simulink model "computedTorquePD"  (R2016a)
settings: Solver=ode45  StartTime=0.0  StopTime=5  RelTol=1e-3
undefined symbols (not defined in the file): ADAMS_cwd, ADAMS_exec, ADAMS_host, ADAMS_init, ADAMS_inputs, ADAMS_outputs, ADAMS_prefix, ADAMS_static, ADAMS_sysdir
settings Model: Creator=admin  LastModifiedBy=Aniket
settings SolverCC: ZeroCrossControl=DisableAll  AlgebraicLoopSolver=LineSearch
settings DataIOCC: LimitDataPoints=on  SaveFormat=Array
settings DebuggingCC: AlgebraicLoopMsg=none
settings HardwareCC: ProdBitPerPointer=32  ProdLargestAtomicFloat=None  ProdIntDivRoundTo=Undefined  ProdEndianess=Unspecified  ProdWordSize=32  ProdHWDeviceType=32-bit Generic
settings ModelReferenceCC: PropagateSignalLabelsOutOfModel=off
settings ConfigComp: CovModelRefEnable=Off

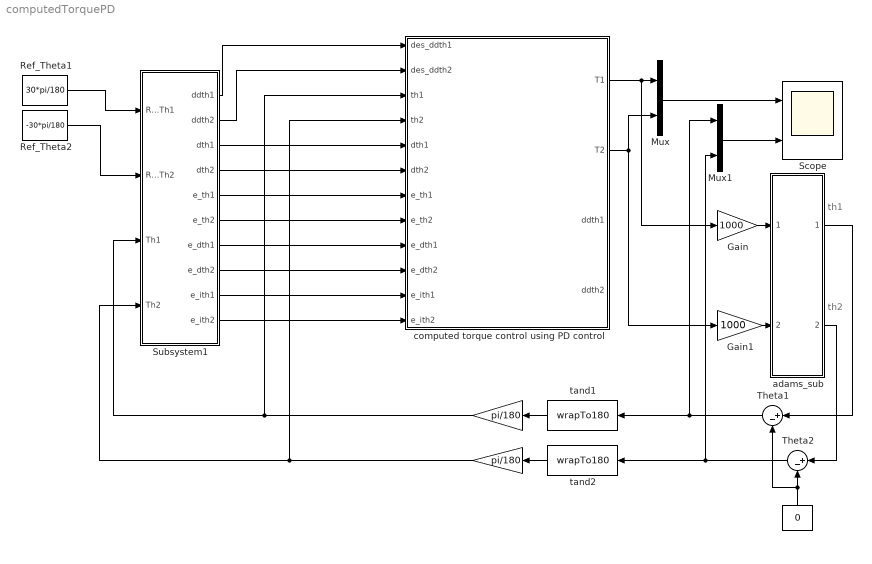
== system computedTorquePD ==
  note: th1
  note: th2
  " " : Constant  Value=0  SampleTime=-1
  "  " : Gain  Gain=pi/180
  "   " : Gain  Gain=pi/180
  Gain : Gain  Gain=1000
  Gain1 : Gain  Gain=1000
  Mux : Mux  Inputs=2
  Mux1 : Mux  Inputs=2
  Ref_Theta1 : Constant  Value=30*pi/180  SampleTime=-1
  Ref_Theta2 : Constant  Value=-30*pi/180  SampleTime=-1
  Scope : Scope  NumInputPorts=2
  Subsystem1 : Subsystem
  Theta1 : Sum  Inputs=|+-
  Theta2 : Sum  Inputs=|+-
  adams_sub : Subsystem
  computed torque control using PD control : MATLAB Function  TreatAsAtomicUnit=on
  tand1 : MATLABFcn  MATLABFcn=wrapTo180
  tand2 : MATLABFcn  MATLABFcn=wrapTo180
  wires:
  Gain/1 -> adams_sub/1("Torque_rear ")
  computed torque control using PD control/1(T1) -> Mux/1, Gain/1
  Ref_Theta1/1 -> Subsystem1/1(Ref_Th1)
  Ref_Theta2/1 -> Subsystem1/2(Ref_Th2)
  Mux/1 -> Scope/1
  computed torque control using PD control/2(T2) -> Mux/2, Gain1/1
  Mux1/1 -> Scope/2
  "  "/1 -> computed torque control using PD control/4(th2), Subsystem1/4(Th2)
  Gain1/1 -> adams_sub/2(Torque_front)
  Theta1/1 -> tand1/1, Mux1/1
  Theta2/1 -> tand2/1, Mux1/2
  adams_sub/2(Theta_front) -> Theta2/1
  adams_sub/1("Theta_rear ") -> Theta1/1
  " "/1 -> Theta1/2, Theta2/2
  tand1/1 -> "   "/1
  tand2/1 -> "  "/1
  "   "/1 -> computed torque control using PD control/3(th1), Subsystem1/3(Th1)
  Subsystem1/1(ddth1) -> computed torque control using PD control/1(des_ddth1)
  Subsystem1/2(ddth2) -> computed torque control using PD control/2(des_ddth2)
  Subsystem1/5(e_th1) -> computed torque control using PD control/7(e_th1)
  Subsystem1/6(e_th2) -> computed torque control using PD control/8(e_th2)
  Subsystem1/7(e_dth1) -> computed torque control using PD control/9(e_dth1)
  Subsystem1/8(e_dth2) -> computed torque control using PD control/10(e_dth2)
  Subsystem1/9(e_ith1) -> computed torque control using PD control/11(e_ith1)
  Subsystem1/10(e_ith2) -> computed torque control using PD control/12(e_ith2)
  Subsystem1/3(dth1) -> computed torque control using PD control/5(dth1)
  Subsystem1/4(dth2) -> computed torque control using PD control/6(dth2)

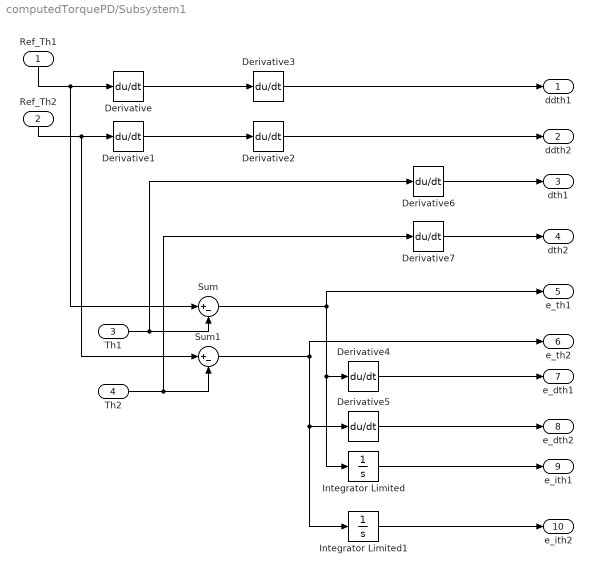
== system computedTorquePD/Subsystem1 ==
  Ref_Th1 : Inport
  Ref_Th2 : Inport  Port=2
  Th1 : Inport  Port=3
  Th2 : Inport  Port=4
  Derivative{,1..3,6..7} (6 alike) : Derivative
  Derivative4 : Derivative  CoefficientInTFapproximation=120
  Derivative5 : Derivative  CoefficientInTFapproximation=120
  Integrator Limited : Integrator  LimitOutput=on
  Integrator Limited1 : Integrator  LimitOutput=on
  Sum : Sum  Inputs=|+-
  Sum1 : Sum  Inputs=|+-
  ddth1 : Outport
  ddth2 : Outport  Port=2
  dth1 : Outport  Port=3
  dth2 : Outport  Port=4
  e_th1 : Outport  Port=5
  e_th2 : Outport  Port=6
  e_dth1 : Outport  Port=7
  e_dth2 : Outport  Port=8
  e_ith1 : Outport  Port=9
  e_ith2 : Outport  Port=10
  wires:
  Derivative3/1 -> ddth1/1
  Derivative2/1 -> ddth2/1
  Derivative/1 -> Derivative3/1
  Ref_Th2/1 -> Sum1/1, Derivative1/1
  Ref_Th1/1 -> Sum/1, Derivative/1
  Derivative1/1 -> Derivative2/1
  Th2/1 -> Derivative7/1, Sum1/2
  Th1/1 -> Derivative6/1, Sum/2
  Sum/1 -> e_th1/1, Derivative4/1, Integrator Limited/1
  Sum1/1 -> e_th2/1, Integrator Limited1/1, Derivative5/1
  Derivative4/1 -> e_dth1/1
  Derivative5/1 -> e_dth2/1
  Integrator Limited/1 -> e_ith1/1
  Integrator Limited1/1 -> e_ith2/1
  Derivative6/1 -> dth1/1
  Derivative7/1 -> dth2/1

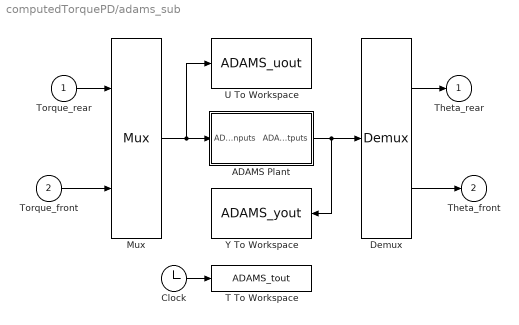
== system computedTorquePD/adams_sub ==
  "Torque_rear " : Inport
  Torque_front : Inport  Port=2
  ADAMS Plant : Subsystem  LoadFcn=|  InitFcn=clear mex  mask(Adams Plant){exevie=ADAMS_sysdir, nam_in=ADAMS_inputs, namout=ADAMS_outputs, nampre=ADAMS_prefix, outfil=ADAMS_prefix, exesol=ADAMS_exec, stat=ADAMS_static, inicmd=[ADAMS_init], exetyp=C++, comtyp=PIPE(DDE), workdir=ADAMS_cwd, ada_host=ADAMS_host, modani=interactive, modsim=discrete, dft=no, simulink_lead_cosim=yes, pin_interp_order=0, pout_extrap_order=0, pin_extrap_order=0, pout_interp_order=0, dt_out=0.005, o_rate=1, more=off}
      | %check based on dialog box setting for when setting by popup menu                                             
      | if exist('ADAMS_solver_type')                                                                                 
      |   if strcmp(ADAMS_solver_type,'C++')                                                                          
      |     set_param(gcb,'exetyp','C++');                                                                            
      |   else                                                                                                        
      |     set_param(gcb,'exetyp','Fortran');                                                                        
      |   end                                                                                                         
      | else                                                                                                          
      |   set_param(gcb,'exetyp','C++');                                                                              
      | end                                                                                                           
      | %set the mode if using acar_solver                                                                            
      | %REQUIRED HERE BECAUSE BELOW CAUSES MDLTERMINATE TO BE CALLED 2 TIMES IN MIDDLE OF SIMULATION WHEN SET IN MASK
      |                                                                                                               
      | %enable the direct feedthrough, sim mode, anim mode parameters by default                                     
      |                                                                                                               
      | if exist('set_some_params_states')                                                                            
      |                                                                                                               
      |   set_some_params_states({'dft','modsim','modani'},{'on','on','on'},'MaskEnables',gcb)                        
      |   %turn on direct feedthrough option                                                                          
      |   set_some_params_states({'dft'},{'on'},'MaskVisibilities',gcb)                                               
      |                                                                                                               
      |  end                                                                                                          
      |                                                                                                               
      |                                                                                                               
      | if exist('ADAMS_exec')                                                                                        
      |   if and(strcmp(get_param(gcb,'exesol'),'ADAMS_exec'),strcmp(ADAMS_exec,'acar_solver'))                       
      |     %set the sim mode to discrete -- only supported mode                                                      
      |     set_param(gcb,'modsim','discrete')                                                                        
      |      %turn off direct feedthrough option                                                                      
      |      set_some_params_states({'dft'},{'off'},'MaskVisibilities',gcb)                                           
      |     %set the animation mode to batch -- only supported mode                                                   
      |     set_param(gcb,'modani','batch')                                                                           
      |     %disable the direct feedthrough, sim mode, anim mode parameters                                           
      |     set_some_params_states({'modsim','modani'},{'off','off'},'MaskEnables',gcb)                               
      |   end                                                                                                         
      | end
      mask prompts: exevie "Adams install directory"; nam_in "Adams View input names"; namout "Adams View output names"; nampre "Adams model file prefix"; outfil "Output files prefix (opt.: if blank - no output)"; exesol "User executable (opt.: if blank - use standard)"; stat "Initial static simulation flag"; inicmd "Initialization commands"; exetyp "Adams Solver type"; comtyp "Interprocess option"; workdir "Adams working directory"; ada_host "Adams host"; modani "Animation mode"; modsim "Simulation mode"; dft "Direct feedthrough"; simulink_lead_cosim "Discrete Computational Order - Simulink Leads Adams"; pin_interp_order "Plant input interpolation order"; pout_extrap_order "Plant output extrapolation order"; pin_extrap_order "Plant input extrapolation order"; pout_interp_order "Plant output interpolation order"; dt_out "Communication interval"; o_rate "Number of communications per output step"; more "More parameters"
      mask help: Simulate any Adams plant model either in Adams Solver form (.adm file) or in Adams View form (.cmd file)
      settings: OpenFcn=|
      | open_system(gcb,'mask')
      | if not(exist('set_some_params_states'))
      | 
      | warning('The script "set_some_params_states.m" cannot be found in the MATLAB PATH.  Cannot update the ADAMS Plant S-Function parameters.')
      | 
      | warning('Recommended action(optional):  run the Adams Controls .m file first to help choose the correct settings in the Adams S-Function block.')
      | 
      | end
      mask Help:
      | <html>
      | This S-Function represents the non-linear Adams Plant with the inputs sent to the Adams model <br>
      |  and the outputs generated by the Adams model.  See the Adams Controls documentation for more <br>
      | information.  This plant uses the following variables:<br>
      | <br>
      | <b>ADAMS_sysdir  :</b> Adams installation directory<br>
      | <b>ADAMS_inputs  :</b> Input variables View names vector<br>
      | <b>ADAMS_outputs :</b> Outputs variables View names vector<br>
      | <b>ADAMS_prefix  : </b>ADAMS model files prefix (.adm, .cmd); also doubles as output files prefix<br>
      | <b>ADAMS_exec :</b> Adams Solver user library or keyword (e.g., acar_solver)<br>
      | <b>ADAMS_static :</b> yes|no - initial static before Co-simulation(discrete)/Function Evaluation(continuous)<br>
      | <b>ADAMS_init :</b>Initialization commands (i.e., Adams View or Solver commands, depending on setting for Animation mode)<br>
      | <b>ADAMS_cwd : </b> Current working directory (for TCP/IP)<br>
      | <b>ADAMS_host : </b>Name of Adams server host (for TCP/IP)<br>
      | <b>ADAMS_mode :</b> Linear or non-linear (i.e., co-sim, function eval)<br>
      | <b>ADAMS_solver_type :</b>Fortran or C++ (used to set popup menu when first loaded) <br>
      | 
      | 
      | <br>
      | The following settings can be chosen:<br>
      | <br>
      | <b>Adams Solver type:</b>  Fortran or C++ (will also set ADAMS_solver_type)<br>
      | <b>Interprocess option:</b> Pipe(DDE) or TCP/IP; TCP/IP can allow different machines run Adams and MATLAB<br>
      | <b>Animation mode:</b> batch (Solver, uses .adm) or interactive (View, uses .cmd)<br>
      | <b>Simulation mode:</b> discrete (Co-simulation) or continuous (Function Evaluation)<br>
      | <b>Discrete Computational Order - Simulink Lead Adams:</b> for discrete mode, chooses if Simulink leads the integration (yes) or lags (no);<br> if set to "no", can remove algebraic loop<br>
      | <b>Plant input interpolation order:</b> 0 = zero-order hold; 1 = linear (discrete mode only, where Simulink leads)<br>
      | <b>Plant output extrapolation order:</b> 0 = zero-order hold;1 = linear(discrete mode only, where Simulink leads)<br>
      | <b>Plant input extrapolation order:</b> 0 = zero-order hold; 1 = linear (discrete mode only, where Adams leads)<br>
      | <b>Plant output interpolation order:</b> 0 = zero-order hold;1 = linear(discrete mode only, where Adams leads)<br>
      | <b>Direct feedthrough:</b> yes|no - yes = Input directly effect output(continuous mode-only)<br>
      | <b>Communication interval:</b> Time step at which Co-simulation exchange information (e.g.,0.005); also controls <br>output for continuous mode (Function Evaluation)<br>
      | <b>Number of communications per output step: </b>Sets Adams output rate (.res, .req, .gra) integer value (default: 1)<br>
      | </html>
      mask Callback exesol:
      | if exist('set_some_params_states')
      | %enable the direct feedthrough, sim mode, anim mode parameters
      | set_some_params_states({'dft','modsim','modani'},{'on','on','on'},'MaskEnables',gcb)
      | %turn on direct feedthrough option
      | set_some_params_states({'dft'},{'on'},'MaskVisibilities',gcb)
      | end
      | 
      | if exist('ADAMS_exec')
      |   if and(strcmp(get_param(gcb,'exesol'),'ADAMS_exec'),strcmp(ADAMS_exec,'acar_solver'))
      |     %set the sim mode to discrete -- only supported mode
      |     %REMOVED:  BELOW CAUSES MDLTERMINATE TO BE CALLED 2 TIMES IN MIDDLE OF SIMULATION
      |     %Now in LoadFcn callback
      |     %set_param(gcb,'modsim','discrete')
      |      %turn off direct feedthrough option
      |     set_some_params_states({'dft'},{'off'},'MaskVisibilities',gcb)
      |     %set the animation mode to batch -- only supported mode
      |     %REMOVED:  BELOW CAUSES MDLTERMINATE TO BE CALLED 2 TIMES IN MIDDLE OF SIMULATION
      |     %Now in LoadFcn callback
      |     %set_param(gcb,'modani','batch')
      |     %disable the direct feedthrough, sim mode, anim mode parameters
      |     set_some_params_states({'modsim','modani'},{'off','off'},'MaskEnables',gcb)
      |   end
      | end
      mask TypeOptions exetyp: Fortran | C++
      mask Callback exetyp:
      | if strcmp(get_param(gcb,'exetyp'),'C++')
      |     ADAMS_solver_type='C++';
      | else
      |     ADAMS_solver_type='Fortran';
      | end
      mask TypeOptions comtyp: PIPE(DDE) | TCP/IP
      mask Callback comtyp:
      | if exist('set_some_params_states')
      | if strcmp(get_param(gcb,'comtyp'),'PIPE(DDE)')
      |     %turn off cwd, host options
      |     set_some_params_states({'ada_host','workdir'},{'off','off'},'MaskVisibilities',gcb)
      | else%if strcmp(get_param(gcb,'modsim'),'TCP/IP')
      |     %turn on cwd, host options
      |     set_some_params_states({'ada_host','workdir'},{'on','on'},'MaskVisibilities',gcb)
      | end
      | end
      mask TypeOptions modani: batch | interactive
      mask TypeOptions modsim: discrete | continuous
      mask Callback modsim:
      | if exist('set_some_params_states')
      | if strcmp(get_param(gcb,'modsim'),'discrete')
      |      %turn off direct feedthrough option
      |     set_some_params_states({'dft'},{'off'},'MaskVisibilities',gcb)
      |     %turn on discrete co-sim type if want to see more
      |     if strcmp(get_param(gcb,'more'),'on')
      |         set_some_params_states({'simulink_lead_cosim'},{'on'},'MaskVisibilities',gcb)
      |     end
      |     if strcmp(get_param(gcb,'simulink_lead_cosim'),'yes')
      |         %turn on interpolation/extrapolation options
      |         set_some_params_states({'pin_interp_order','pout_extrap_order',},{'on','on'},'MaskVisibilities',gcb)
      |     else
      |         set_some_params_states({'pin_extrap_order','pout_interp_order'},{'on','on'},'MaskVisibilities',gcb)
      |     end
      | else%if strcmp(get_param(gcb,'modsim'),'continuous')
      |      %turn off direct feedthrough option
      |     set_some_params_states({'dft'},{'on'},'MaskVisibilities',gcb)
      |     %turn off interpolation/extrapolation options
      |     set_some_params_states({'pin_interp_order','pout_extrap_order','pin_extrap_order','pout_interp_order','simulink_lead_cosim'},{'off','off','off','off','off'},'MaskVisibilities',gcb)
      | end
      | end
      mask TypeOptions dft: no | yes
      mask TypeOptions simulink_lead_cosim: yes | no
      mask Callback simulink_lead_cosim:
      | if exist('set_some_params_states')
      | if (strcmp(get_param(gcb,'simulink_lead_cosim'),'yes') && strcmp(get_param(gcb,'modsim'),'discrete'))
      |      %turn off unused interpolate/extrapolate options
      |     set_some_params_states({'pin_extrap_order','pout_interp_order'},{'off','off'},'MaskVisibilities',gcb)
      |     %turn on used interpolate/extrapolate options
      |     set_some_params_states({'pin_interp_order','pout_extrap_order'},{'on','on'},'MaskVisibilities',gcb)
      | elseif (strcmp(get_param(gcb,'simulink_lead_cosim'),'no') && strcmp(get_param(gcb,'modsim'),'discrete'))
      |     %turn on used interpolate/extrapolate options
      |     set_some_params_states({'pin_extrap_order','pout_interp_order'},{'on','on'},'MaskVisibilities',gcb)
      |      %turn off unused interpolate/extrapolate options
      |     set_some_params_states({'pin_interp_order','pout_extrap_order'},{'off','off'},'MaskVisibilities',gcb)
      | end
      | end
      mask TypeOptions pin_interp_order: 0 | 1
      mask TypeOptions pout_extrap_order: 0 | 1
      mask TypeOptions pin_extrap_order: 0 | 1
      mask TypeOptions pout_interp_order: 0 | 1
      mask Callback more:
      | if exist('set_some_params_states')
      | if (strcmp(get_param(gcb,'more'),'on'))
      |      %turn on infrequently used options
      |     set_some_params_states({'exevie','nam_in','namout','exesol','stat','inicmd'},{'on','on','on','on','on','on'},'MaskVisibilities',gcb)
      |     if strcmp(get_param(gcb,'modsim'),'discrete')
      |         set_some_params_states({'simulink_lead_cosim'},{'on'},'MaskVisibilities',gcb)
      |     end
      | elseif (strcmp(get_param(gcb,'more'),'off'))
      |     %turn off infrequently used options
      |     set_some_params_states({'exevie','nam_in','namout','exesol','stat','inicmd'},{'off','off','off','off','off','off'},'MaskVisibilities',gcb)
      |     if strcmp(get_param(gcb,'modsim'),'discrete')
      |         set_some_params_states({'simulink_lead_cosim'},{'off'},'MaskVisibilities',gcb)
      |     end
      | end
      | end
      mask Display: disp( 'MSC Software' )
  Clock : Clock
  Demux : Demux  Outputs=2
  Mux : Mux  Inputs=2
  T To Workspace : ToWorkspace  VariableName=ADAMS_tout
      settings: MaxDataPoints=100000
  U To Workspace : ToWorkspace  VariableName=ADAMS_uout
      settings: MaxDataPoints=100000
  Y To Workspace : ToWorkspace  VariableName=ADAMS_yout
      settings: MaxDataPoints=100000
  "Theta_rear " : Outport
  Theta_front : Outport  Port=2
  wires:
  Clock/1 -> T To Workspace/1
  Mux/1 -> ADAMS Plant/1(ADAMS inputs), U To Workspace/1
  ADAMS Plant/1(ADAMS outputs) -> Demux/1, Y To Workspace/1
  Demux/1 -> "Theta_rear "/1
  Demux/2 -> Theta_front/1
  "Torque_rear "/1 -> Mux/1
  Torque_front/1 -> Mux/2

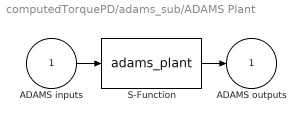
== system computedTorquePD/adams_sub/ADAMS Plant ==
  ADAMS inputs : Inport
  S-Function : S-Function  StopFcn=clear mex  FunctionName=adams_plant  Parameters=exevie,exesol,stat,outfil,nampre,o_rate,nam_in,namout,dft,modsim,modani,dt_out,inicmd,exetyp,comtyp,ada_host, workdir,pin_interp_order,pout_extrap_order,pin_extrap_order,pout_interp_order,simulink_lead_cosim  SFunctionDeploymentMode=off  EnableBusSupport=off
  ADAMS outputs : Outport  InitialOutput=0
  wires:
  ADAMS inputs/1 -> S-Function/1
  S-Function/1 -> ADAMS outputs/1

== matlab function computedTorquePD/computed torque control using PD control ==
  data: T1 output; des_ddth1 input; des_ddth2 input; T2 output; ddth1 output; ddth2 output; th1 input; th2 input; dth1 input; dth2 input; e_th1 input; e_th2 input; e_dth1 input; e_dth2 input; e_ith1 input; e_ith2 input
function [T1,T2,ddth1,ddth2]    = fcn1(des_ddth1,des_ddth2,th1,th2,...
                                        dth1,dth2,e_th1,e_th2,e_dth1,...
                                        e_dth2,e_ith1,e_ith2)
%computed torque control method PD control
a1 = 0.40 ; a2 = 0.35; m1 = 0.1287; m2 = 0.1024; g = 9.8;

Kp = 500*diag([1 1.2],0);
Kd = 0*diag([1 1],0);             %for critical damping & Filter_Coeff = 100 
Ki = 50*diag([1 10],0);

D = [ ((a1^2*m1)/3 + a1^2*m2 + (a2^2*m2)/3)*ones + a1*a2*m2*cos(th2), (m2*a2^2)/3 + (a1*m2*cos(th2)*a2)/2;
                     (m2*a2^2)/3 + (a1*m2*cos(th2)*a2)/2,                            (a2^2*m2)/3];
H = [ -(a1*a2*m2*sin(th2)*(2*dth1 + dth2)*dth2)/2;
                                      (a1*a2*m2*sin(th2)*dth1^2)/2];
C = [ (a2*g*m2*cos(th1 + th2))/2 + (a1*g*m1*cos(th1))/2 + a1*g*m2*cos(th1);
                                                 (a2*g*m2*cos(th1 + th2))/2];

e = [e_th1;e_th2;e_dth1;e_dth2;e_ith1;e_ith2];
u = -Kd*[e(3);e(4)]-Kp*[e(1);e(2)]-Ki*[e(5);e(6)];
U = D*([des_ddth1;des_ddth2]-u)+H+C;
T1 = U(1);
T2 = U(2);
ddt = inv(D)*(U-H-C);
ddth1 = ddt(1);
ddth2 = ddt(2);
